simulink model "Lineal_Model_quadrotor"  (R2023a)
settings: Solver=VariableStepAuto  StartTime=0.0  StopTime=10.0  RelTol=1e-3
undefined symbols (not defined in the file): A, B, C, K
settings Model: Creator=jonat  LastModifiedBy=jonat

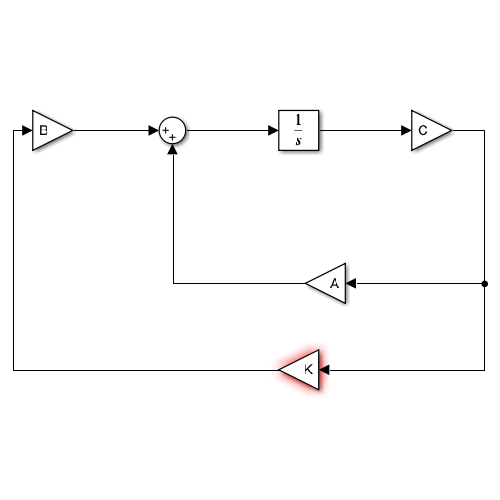
[thumbnail: Simulink's stored preview of the top-level diagram]
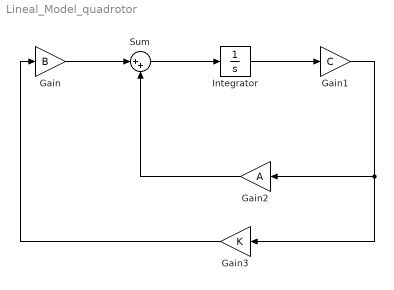
== system Lineal_Model_quadrotor ==
  Gain : Gain  Gain=B
  Gain1 : Gain  Gain=C
  Gain2 : Gain  Gain=A
  Gain3 : Gain  Gain=K
  Integrator : Integrator
  Sum : Sum  Inputs=|++
  wires:
  Integrator/1 -> Gain1/1
  Gain/1 -> Sum/1
  Sum/1 -> Integrator/1
  Gain2/1 -> Sum/2
  Gain3/1 -> Gain/1
  Gain1/1 -> Gain3/1, Gain2/1
